simulink model "F550_model_trim_ver2023b"  (R2023b)
settings: Solver=ode4  StartTime=0.0  StopTime=100  FixedStep=0.001  RelTol=1e-3
undefined symbols (not defined in the file or in its folder): u0
settings Model: Creator=ADMIN  LastModifiedBy=CNU_UASG
settings DataIOCC: ExternalInput=getinputstruct(op_trim3)  InitialState=getstatestruct(op_trim3)
settings DebuggingCC: UnconnectedInputMsg=warning  UnconnectedOutputMsg=warning  UnconnectedLineMsg=warning
settings ModelReferenceCC: EnableRefExpFcnMdlSchedulingChecks=on
settings RTWCC: DLArmComputeVersion=19.05

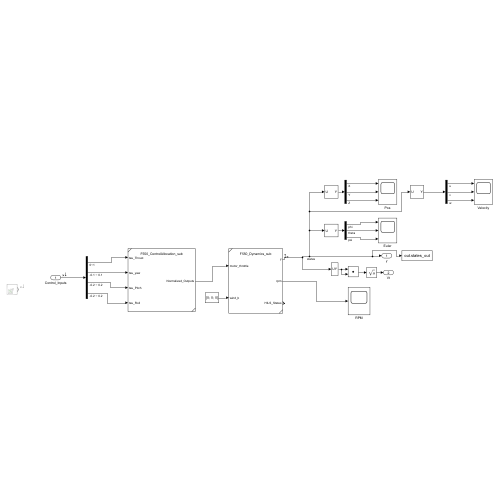
[thumbnail: Simulink's stored preview of the top-level diagram]
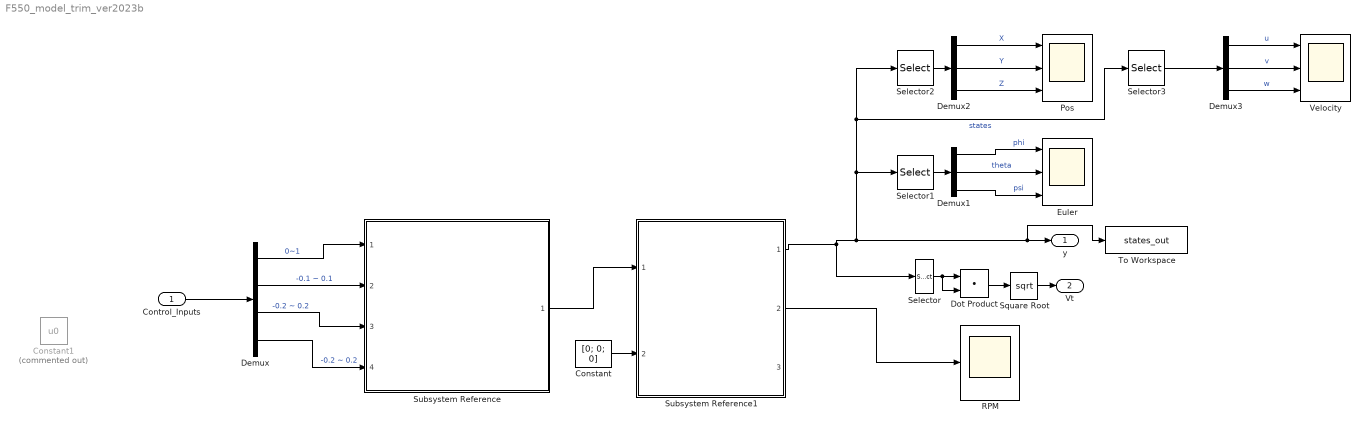
== system F550_model_trim_ver2023b ==
  Control_Inputs : Inport
  Constant : Constant  Value=[0; 0; 0]
  Constant1 : Constant  Commented=on  Value=u0
  Demux : Demux
  Demux1 : Demux  Outputs=3
  Demux2 : Demux  Outputs=3
  Demux3 : Demux  Outputs=3
  Dot Product : DotProduct  OutDataTypeStr=Inherit: Inherit via internal rule
  Euler : Scope  NumInputPorts=3
  Pos : Scope  NumInputPorts=3
  RPM : Scope
  Selector : Selector  InputPortWidth=12  IndexOptions=Index vector (dialog)  Indices=[1 2 3]  OutputSizes=1
  Selector1 : Selector  InputPortWidth=12  IndexOptions=Index vector (dialog)  Indices=[7 8 9]  OutputSizes=1
  Selector2 : Selector  InputPortWidth=12  IndexOptions=Index vector (dialog)  Indices=[ 10 11 12]  OutputSizes=1
  Selector3 : Selector  InputPortWidth=12  IndexOptions=Index vector (dialog)  Indices=[1 2 3]  OutputSizes=1
  Square Root : Sqrt
  Subsystem Reference : Subsystem  ReferencedSubsystem=F550_ControlAllocation_sub
  Subsystem Reference1 : Subsystem  ReferencedSubsystem=F550_Dynamics_sub
  To Workspace : ToWorkspace  VariableName=states_out  SampleTime=-1
  Velocity : Scope  NumInputPorts=3
  y : Outport
  Vt : Outport  Port=2
  wires:
  Demux/4 -> Subsystem Reference/4  "-0.2 ~ 0.2"
  Demux/3 -> Subsystem Reference/3  "-0.2 ~ 0.2"
  Demux/2 -> Subsystem Reference/2  "-0.1 ~ 0.1"
  Demux/1 -> Subsystem Reference/1  "0~1"
  Subsystem Reference1/2 -> RPM/1
  Selector/1 -> Dot Product/1, Dot Product/2
  Square Root/1 -> Vt/1
  Dot Product/1 -> Square Root/1
  Subsystem Reference1/1 -> Selector/1, Selector3/1, Selector2/1, Selector1/1, To Workspace/1, y/1  "states"
  Constant/1 -> Subsystem Reference1/2
  Subsystem Reference/1 -> Subsystem Reference1/1
  Selector1/1 -> Demux1/1
  Demux1/1 -> Euler/1  "phi"
  Demux1/2 -> Euler/2  "theta"
  Demux1/3 -> Euler/3  "psi"
  Demux2/1 -> Pos/1  "X"
  Demux2/2 -> Pos/2  "Y"
  Demux2/3 -> Pos/3  "Z"
  Selector2/1 -> Demux2/1
  Demux3/3 -> Velocity/3  "w"
  Selector3/1 -> Demux3/1
  Demux3/2 -> Velocity/2  "v"
  Demux3/1 -> Velocity/1  "u"
  Control_Inputs/1 -> Demux/1
